simulink model "Quartenion"  (R2018b)
settings: Solver=VariableStepAuto  StartTime=0.0  StopTime=10.0  RelTol=1e-3
values from neighbouring files (symbols this model uses):
  A = [exp(-delT/tcons) zeros(1,6) ... (first row only)    [EKF.m]
  delT = 0.001    [EKF.m]
  H = I    [EKF.m]
  K = pmin*H'*(H*pmin*H'+R)    [EKF.m]
  tcons = 0.5    [EKF.m]
  varW = 0.4    [EKF.m]
  xinit = [ones(1,7)]'    [EKF.m]
libraries: simulink x1, dspsrcs4 x1, aerolibutil x1
settings Model: Creator=ASUS  LastModifiedBy=ASUS

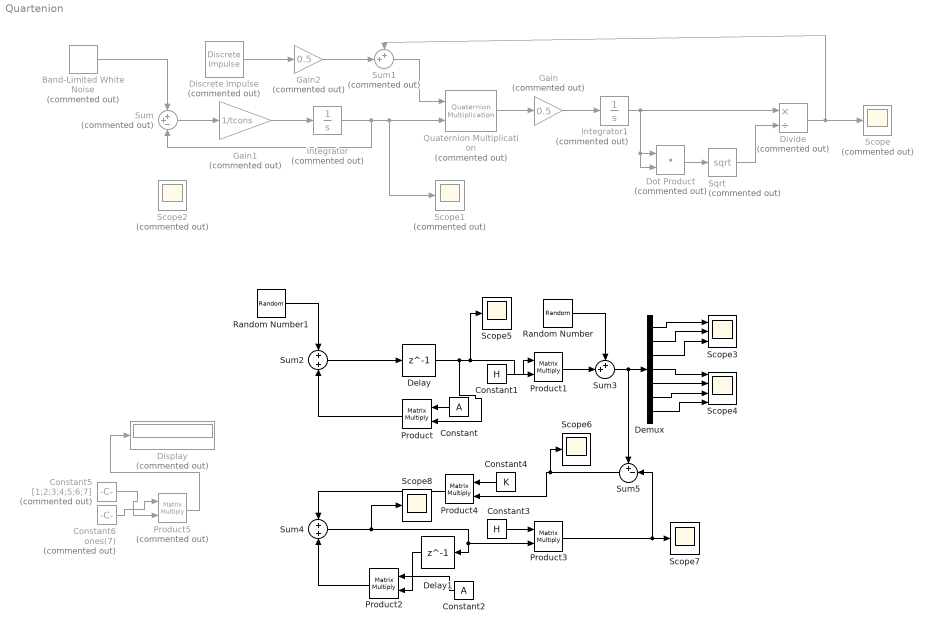
== system Quartenion ==
  Band-Limited White Noise : simulink/Sources/Band-Limited White Noise  Commented=on  Cov=[0; 0.1;0.1;0.1]  Ts=0.1  seed=[0 23340 23341 23342]
  Constant : Constant  Value=A
  Constant1 : Constant  Value=H
  Constant2 : Constant  Value=A
  Constant3 : Constant  Value=H
  Constant4 : Constant  Value=K
  Constant5 : Constant  Commented=on  Value=[1;2;3;4;5;6;7]
  Constant6 : Constant  Commented=on  Value=ones(7)
  Delay : Delay  DelayLength=1  InitialCondition=xinit
  Delay1 : Delay  DelayLength=1  InitialCondition=xinit
  Demux : Demux  Outputs=7
  Discrete Impulse : dspsrcs4/Discrete  Impulse  Commented=on  Delay=[0 0 0 0]  SampleTime=delT  FrameSample=1  OutputFrames=off  dataType=double  isSigned=on  wordLen=16  udDataType=sfix(16)  fracBitsMode=Best precision  numFracBits=15  OutDataTypeStr=double  LastOutDataTypeStr=double
  Display : Display  Commented=on
  Divide : Product  Commented=on  Inputs=*/
  Dot Product : DotProduct  Commented=on  InputSameDT=on  OutDataTypeStr=Inherit: Inherit via internal rule
  Gain : Gain  Commented=on  Gain=0.5
  Gain1 : Gain  Commented=on  Gain=1/tcons
  Gain2 : Gain  Commented=on  Gain=0.5
  Integrator : Integrator  Commented=on
  Integrator1 : Integrator  Commented=on  InitialCondition=0.1
  Product{,1..4} (5 alike) : Product  Multiplication=Matrix(*)
  Product5 : Product  Commented=on  Multiplication=Matrix(*)
  Quaternion Multiplication : aerolibutil/Quaternion Multiplication  Commented=on
  Random Number : RandomNumber  Mean=[0 0 0 0 0 0 0]  Variance=[0.01 0.01 0.01 0.0001 0.0001 0.0001 0.0001]  Seed=[1 2 3 4 5 6 7]  SampleTime=delT
  Random Number1 : RandomNumber  Mean=[0 0 0 0 0 0 0]  Variance=[varW varW varW 0 0 0 0]  Seed=[1 2 3 4 5 6 7]  SampleTime=delT
  Scope : Scope  Commented=on
  Scope1 : Scope  Commented=on
  Scope2 : Scope  Commented=on
  Scope3 : Scope  NumInputPorts=3
  Scope4 : Scope  NumInputPorts=4
  Scope{5..8} (4 alike) : Scope
  Sqrt : Sqrt  Commented=on  SaturateOnIntegerOverflow=on
  Sum : Sum  Commented=on  Inputs=++-
  Sum1 : Sum  Commented=on  Inputs=++|
  Sum2 : Sum  Inputs=+|+
  Sum3 : Sum  Inputs=++|
  Sum4 : Sum  Inputs=+|+
  Sum5 : Sum  Inputs=+-|
  wires:
  Quaternion Multiplication/1 -> Gain/1
  Gain1/1 -> Integrator/1
  Sum/1 -> Gain1/1
  Band-Limited White Noise/1 -> Sum/1
  Gain/1 -> Integrator1/1
  Integrator1/1 -> Dot Product/2, Dot Product/1, Divide/1
  Discrete Impulse/1 -> Gain2/1
  Gain2/1 -> Sum1/2
  Sum1/1 -> Quaternion Multiplication/1
  Dot Product/1 -> Sqrt/1
  Sqrt/1 -> Divide/2
  Divide/1 -> Sum1/1, Scope/1
  Integrator/1 -> Sum/3, Scope1/1, Quaternion Multiplication/2
  ? -> Scope2/1, Sum/2
  Constant/1 -> Product/1
  Constant1/1 -> Product1/1
  Delay/1 -> Product/2, Product1/2, Scope5/1
  Sum2/1 -> Delay/1
  Product/1 -> Sum2/2
  Random Number1/1 -> Sum2/1
  Random Number/1 -> Sum3/1
  Product1/1 -> Sum3/2
  Sum3/1 -> Sum5/1, Demux/1
  Demux/1 -> Scope3/1
  Demux/2 -> Scope3/2
  Demux/3 -> Scope3/3
  Demux/4 -> Scope4/1
  Demux/5 -> Scope4/2
  Demux/6 -> Scope4/3
  Demux/7 -> Scope4/4
  Product3/1 -> Scope7/1, Sum5/2
  Constant3/1 -> Product3/1
  Product2/1 -> Sum4/2
  Sum4/1 -> Scope8/1, Delay1/1, Product3/2
  Constant2/1 -> Product2/1
  Product4/1 -> Sum4/1
  Sum5/1 -> Scope6/1, Product4/2
  Constant4/1 -> Product4/1
  Delay1/1 -> Product2/2
  Constant5/1 -> Product5/2
  Constant6/1 -> Product5/1
  Product5/1 -> Display/1
